simulink model "simulink"  (R2024b)
settings: Solver=VariableStepAuto  StartTime=0.0  StopTime=2  RelTol=1e-3
libraries: spsRMSLib x3, spsVoltageMeasurementLib x3, spsDCVoltageSourceLib x1, spsAsynchronousMachineSIUnitsLib x1, spsIdealSwitchLib x1, spsPWMGenerator2LevelLib x1, spsThreePhaseFaultLib x1, spsUniversalBridgeLib x1, sps_lib x1
settings Model: Creator=BHAVE  LastModifiedBy=BHAVE

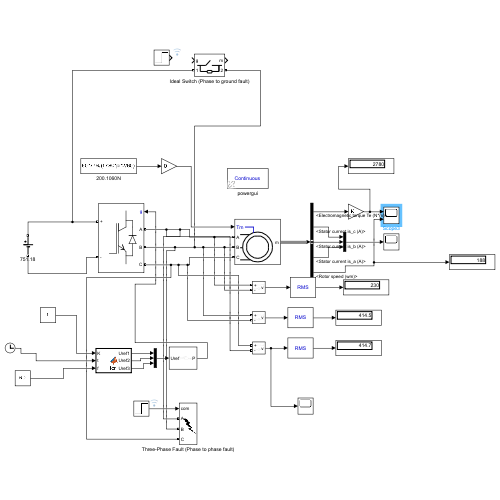
[thumbnail: Simulink's stored preview of the top-level diagram]
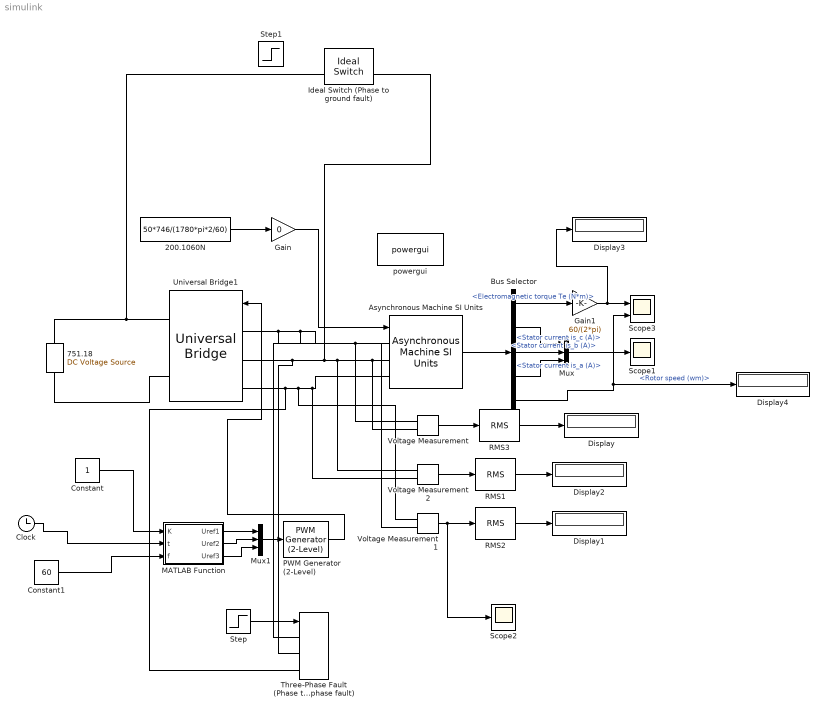
== system simulink ==
  200.1060N : Constant  Value=50*746/(1780*pi*2/60)
  751.18 : spsDCVoltageSourceLib/DC Voltage Source  Amplitude=460/sqrt(3)*sqrt(2)*2  Measurements=None
  Asynchronous Machine SI Units : spsAsynchronousMachineSIUnitsLib/Asynchronous Machine SI Units  RotorType=Squirrel-cage  PresetModel="04:  50 HP  460 V 60Hz 1780 RPM"  MechanicalLoad=Torque Tm  ShowDetailedParameters=on  ReferenceFrame=Rotor  Units=SI  MeasurementBus=off  NominalParameters=[3.73e+04 460 60]  VoltageRatio=1  Stator=[0.09961 0.000867]  Rotor=[0.05837 0.000867]  Cage1=[0.4155 0.002066]  Cage2=[0.4168 0.0003495]  Lm=0.03039  Mechanical=[0.4 0.02187 2]  PolePairs=2  InitialConditions=[1 0 0 0 0 0 0 0]  SimulateSaturation=off  Saturation=[14.03593122, 27.81365428, 53.79336849, 72.68890987, 97.98006896, 148.6815601, 215.7428561, 302.9841135, 428.7778367 ; 230, 322, 414, 460, 506, 552, 598, 644, 690]  LoadFlowParameters=1492000  TsPowergui=0  TsBlock=-1  IterativeModel=Trapezoidal non iterative  IterativeDiscreteModel=Trapezoidal non iterative  Pmec=1.492e+006
  Bus Selector : BusSelector  OutputSignals=Mechanical.Electromagnetic torque Te (N*m),Stator measurements.Stator current is_c (A),Stator measurements.Stator current is_b (A),Stator measurements.Stator current is_a (A),Mechanical.Rotor speed (wm)
  Clock : Clock
  Constant : Constant
  Constant1 : Constant  Value=60
  Display{,1..4} (5 alike) : Display
  Gain : Gain  Gain=0
  Gain1 : Gain  Gain=60/(2*pi)
  Ideal Switch (Phase to ground fault) : spsIdealSwitchLib/Ideal Switch  Ron=1  Lon=0  IC=0  Rs=1e6  Cs=inf  Measurements=on
  MATLAB Function : MATLAB Function  TreatAsAtomicUnit=on
  Mux : Mux  Inputs=3
  Mux1 : Mux  Inputs=3
  PWM Generator (2-Level) : spsPWMGenerator2LevelLib/PWM Generator (2-Level)  ModulatorType=Three-phase bridge (6 pulses)  ModulatorMode=Unsynchronized  Fc=200*60  Pc=90  nF=27  MinMax="[ -1  1 ]"  SamplingTechnique=Natural  ModulatingSignals=off  m=0.8  Freq=60  Phase=0  Ts=0  ShowCarrierOutport=off
  RMS1 : spsRMSLib/RMS  TrueRMS=off  Freq=60  RMSInit=120  Ts=0
  RMS2 : spsRMSLib/RMS  TrueRMS=off  Freq=60  RMSInit=120  Ts=0
  RMS3 : spsRMSLib/RMS  TrueRMS=off  Freq=60  RMSInit=120  Ts=0
  Scope1 : Scope
  Scope2 : Scope
  Scope3 : Scope  NumInputPorts=2
  Step : Step  SampleTime=10e-6
  Step1 : Step  Time=0.5  SampleTime=10e-6
  Three-Phase Fault (Phase to phase fault) : spsThreePhaseFaultLib/Three-Phase Fault  InitialStates=0  FaultA=on  FaultB=on  FaultC=off  GroundFault=off  SwitchTimes="[1/60  5/60]"  External=on  SwitchStatus=NaN  FaultResistance=0.001  GroundResistance=0.001  SnubberResistance=1e6  SnubberCapacitance=inf  Measurements=None
  Universal Bridge1 : spsUniversalBridgeLib/Universal Bridge  Arms=3  SnubberResistance=1e5  SnubberCapacitance=inf  Device=IGBT / Diodes  Ron=1e-3  Lon=0  ForwardVoltages="[  0  0  ]"  ForwardVoltage=0  GTOparameters=[ 10e-6 , 20e-6 ]  IGBTparameters=[ 1e-6 , 2e-6 ]  Measurements=None  Measurements_2=None  converterType=Rectifier
  Voltage Measurement : spsVoltageMeasurementLib/Voltage Measurement  PhasorSimulation=off  OutputType=Complex  PSBequivalent=0
  Voltage Measurement1 : spsVoltageMeasurementLib/Voltage Measurement  PhasorSimulation=off  OutputType=Complex  PSBequivalent=0
  Voltage Measurement2 : spsVoltageMeasurementLib/Voltage Measurement  PhasorSimulation=off  OutputType=Complex  PSBequivalent=0
  powergui : sps_lib/powergui  Priority=1  SimulationMode=Continuous  SampleTime=50e-6  frequency=60  Iterations=50  frequencyindice=60  Pbase=100e6  ErrMax=1e-4  UnitsV=kV  UnitsW=MW  buscounter=0  FunctionMessages=off  echomessages=off  EnableUseOfTLC=off  CurrentSourceSwitches=off  DisableSnubberDevices=off  DisableRonSwitches=off  DisableVfSwitches=off  DisplayEquations=off  AutomaticDiscreteSolvers=off  SolverType=Tustin/Backward Euler (TBE)  Interpol=off  ExternalGateDelay=off  methode=off  Ts=100  x0status=blocks  SPID=on  SwTol=0  HookPort=off  NonlinearTolerance=1e-4  nMaxIteration=100  ContinueOnMaxIteration=off  RestoreLinks=warning  ResistiveCurrentMeasurement=off  Frange=[0:2:500]  Ylog=off  Xlog=on  ShowGrid=off  save=off  variable=ZData  structure=0  ZoomFFT=off  StartTime=0.0  cycles=1  DisplayStyle=1  fundamental=60  FreqAxis=off  MaxFrequency=1000  frequencyindicesteady=1  RmsSteady=1  display=off
  wires:
  200.1060N/1 -> Gain/1
  Gain/1 -> Asynchronous Machine SI Units/1
  Asynchronous Machine SI Units/1 -> Bus Selector/1
  Bus Selector/1 -> Gain1/1  "<Electromagnetic torque Te (N*m)>"
  Bus Selector/5 -> Scope3/2, Display4/1  "<Rotor speed (wm)>"
  Bus Selector/3 -> Mux/2  "<Stator current is_b (A)>"
  Bus Selector/2 -> Mux/1  "<Stator current is_c (A)>"
  Bus Selector/4 -> Mux/3  "<Stator current is_a (A)>"
  Mux/1 -> Scope1/1
  Gain1/1 -> Scope3/1, Display3/1
  PWM Generator (2-Level)/1 -> Universal Bridge1/1
  Mux1/1 -> PWM Generator (2-Level)/1
  MATLAB Function/1(Uref1) -> Mux1/1
  MATLAB Function/2(Uref2) -> Mux1/2
  MATLAB Function/3(Uref3) -> Mux1/3
  Constant/1 -> MATLAB Function/1(K)
  Clock/1 -> MATLAB Function/2(t)
  Constant1/1 -> MATLAB Function/3(f)
  Voltage Measurement/1 -> RMS3/1
  RMS3/1 -> Display/1
  Voltage Measurement2/1 -> RMS1/1
  RMS1/1 -> Display2/1
  RMS2/1 -> Display1/1
  Voltage Measurement1/1 -> Scope2/1, RMS2/1
  Step/1 -> Three-Phase Fault (Phase to phase fault)/1
  connections:
  Universal Bridge1/LConn2 -- Three-Phase Fault (Phase to phase fault)/LConn2 -- Voltage Measurement2/LConn1 -- Voltage Measurement/LConn2 -- Asynchronous Machine SI Units/LConn2 -- Ideal Switch (Phase to ground fault)/RConn1
  751.18/LConn1 -- Universal Bridge1/RConn2
  751.18/RConn1 -- Ideal Switch (Phase to ground fault)/LConn1 -- Universal Bridge1/RConn1
  Universal Bridge1/LConn3 -- Three-Phase Fault (Phase to phase fault)/LConn3 -- Voltage Measurement1/LConn1 -- Voltage Measurement2/LConn2 -- Asynchronous Machine SI Units/LConn3
  Universal Bridge1/LConn1 -- Voltage Measurement1/LConn2 -- Three-Phase Fault (Phase to phase fault)/LConn1 -- Voltage Measurement/LConn1 -- Asynchronous Machine SI Units/LConn1

== matlab function simulink/MATLAB Function ==
  data: K input; Uref1 output; Uref2 output; Uref3 output; t input; f input
function [Uref1,Uref2,Uref3]=fcn(K,t,f)
Uref1=K*sin(2*pi*f*t*K);
Uref2=K*sin(2*pi*f*t*K-2*pi/3);
Uref3=K*sin(2*pi*f*t*K+2*pi/3);
end
